simulink model "Motor_Lag_Controller"  (R2023a)
settings: Solver=ode4  StartTime=0.0  StopTime=3  FixedStep=0.001  RelTol=1e-3
settings Model: Creator=Fasih  LastModifiedBy=Fasih

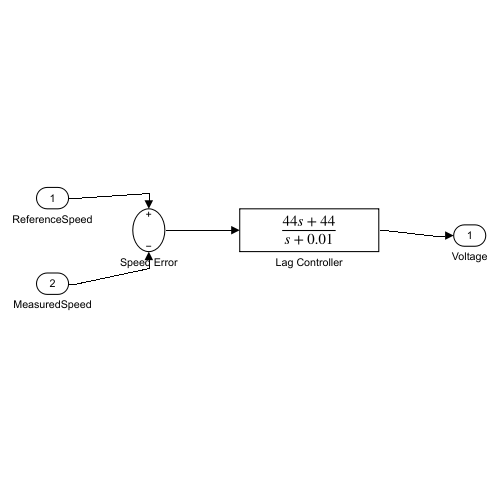
[thumbnail: Simulink's stored preview of the top-level diagram]
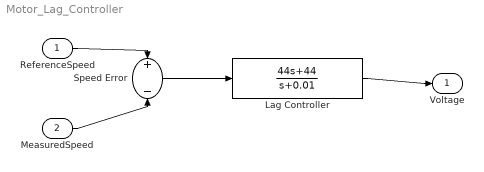
== system Motor_Lag_Controller ==
  ReferenceSpeed : Inport
  MeasuredSpeed : Inport  Port=2
  Lag Controller : TransferFcn  Numerator=[44 44]  Denominator=[1 0.01]
  Speed Error : Sum  Inputs=+-
  Voltage : Outport
  wires:
  ReferenceSpeed/1 -> Speed Error/1
  MeasuredSpeed/1 -> Speed Error/2
  Speed Error/1 -> Lag Controller/1
  Lag Controller/1 -> Voltage/1
